simulink model "mcb_pmsm_foc_sensorless_f28379d1"  (R2026a)
settings: Solver=FixedStepDiscrete  StopTime=8  EnableMultiTasking=on
InitFcn:
  | mcb_pmsm_foc_sensorless_f28379d_datascript;
  | mcb_pmsm_foc_sensorless_f28379d_pi_recovery;
  | mcb_pmsm_foc_sensorless_f28379d_fado_init;
  | mcb_pmsm_foc_sensorless_f28379d_fado_tuning;
  | mcb_pmsm_foc_sensorless_f28379d_fado_testprofile_init;
model workspace (MAT data in the model file):
  encoderResolution = 2000
  hallOffset = '0.5'
  indexOffset = 850
  polePairs = '4'
values from neighbouring files (symbols this model uses):
  acceleration = 10000/PU_System.N_base    [mcb_pmsm_foc_sensorless_f28379d_datascript.m]
  dataType = 'single'    [mcb_pmsm_foc_sensorless_f28379d_datascript.m]
  fado_EnableIdAssist = double(fado.EnableIdAssist)    [mcb_pmsm_foc_sensorless_f28379d_fado_init.m]
  fado_EnableVoltagePreprocess = double(fado.EnableVoltagePreprocess)    [mcb_pmsm_foc_sensorless_f28379d_fado_init.m]
  fado_FluxLimit = fado.FluxLimit    [mcb_pmsm_foc_sensorless_f28379d_fado_init.m]
  fado_IBase = fado.IBase    [mcb_pmsm_foc_sensorless_f28379d_fado_init.m]
  fado_IminPU = fado.IminPU    [mcb_pmsm_foc_sensorless_f28379d_fado_init.m]
  fado_Kaf = fado.Kaf    [mcb_pmsm_foc_sensorless_f28379d_fado_init.m]
  fado_Kdf = fado.Kdf    [mcb_pmsm_foc_sensorless_f28379d_fado_init.m]
  fado_LowSpeedHz = fado.LowSpeedHz    [mcb_pmsm_foc_sensorless_f28379d_fado_init.m]
  fado_Lq = fado.Lq    [mcb_pmsm_foc_sensorless_f28379d_fado_init.m]
  fado_LqEstScale = fado.LqEstScale    [mcb_pmsm_foc_sensorless_f28379d_fado_init.m]
  fado_NBase = fado.NBase    [mcb_pmsm_foc_sensorless_f28379d_fado_init.m]
  fado_PolePairs = fado.PolePairs    [mcb_pmsm_foc_sensorless_f28379d_fado_init.m]
  fado_Rs = fado.Rs    [mcb_pmsm_foc_sensorless_f28379d_fado_init.m]
  fado_RsEstScale = fado.RsEstScale    [mcb_pmsm_foc_sensorless_f28379d_fado_init.m]
  fado_T2SFastBandwidthHz = fado.T2SFastBandwidthHz    [mcb_pmsm_foc_sensorless_f28379d_fado_init.m]
  fado_T2SSlowBandwidthHz = fado.T2SSlowBandwidthHz    [mcb_pmsm_foc_sensorless_f28379d_fado_init.m]
  fado_Ts = fado.Ts    [mcb_pmsm_foc_sensorless_f28379d_fado_init.m]
  fado_VAlphaPreprocess = fado.VAlphaPreprocess    [mcb_pmsm_foc_sensorless_f28379d_fado_init.m]
  fado_VBase = fado.VBase    [mcb_pmsm_foc_sensorless_f28379d_fado_init.m]
  fado_VBetaPreprocess = fado.VBetaPreprocess    [mcb_pmsm_foc_sensorless_f28379d_fado_init.m]
  fado_Zeta = fado.Zeta    [mcb_pmsm_foc_sensorless_f28379d_fado_init.m]
  inverter = mcb.updateInverterParameters(pmsm,inverter,target)    [mcb_pmsm_foc_sensorless_f28379d_datascript.m]
  MAX_OL_NEG_SPD = -0.2    [mcb_pmsm_foc_sensorless_f28379d_datascript.m]
  MAX_OL_POS_SPD = 0.2    [mcb_pmsm_foc_sensorless_f28379d_datascript.m]
  MAX_OL_VD_LIMIT = 0.6    [mcb_pmsm_foc_sensorless_f28379d_datascript.m]
  MIN_CL_NEG_SPD = -0.15    [mcb_pmsm_foc_sensorless_f28379d_datascript.m]
  MIN_CL_POS_SPD = 0.15    [mcb_pmsm_foc_sensorless_f28379d_datascript.m]
  MIN_OL_VD_LIMIT = 0.15    [mcb_pmsm_foc_sensorless_f28379d_datascript.m]
  one_sec_tick = uint16(1/Ts_speed)    [mcb_pmsm_foc_sensorless_f28379d_datascript.m]
  PI_params = mcb.calcFOCGains(motor,Ts,Ts_speed,Base=PU_System,PositionObserver=EEMF,SLFeedbackPathDelay=EEMFSLDelay)    [mcb_pmsm_foc_sensorless_f28379d_datascript.m]
  pmsm = mcb.getPMSMParameters('Teknic2310P')    [mcb_pmsm_foc_sensorless_f28379d_datascript.m]
  PU_System = mcb.getPUSystemParameters(pmsm,inverter)    [mcb_pmsm_foc_sensorless_f28379d_datascript.m]
  RAMP_STEP_SIZE = 0.001    [mcb_pmsm_foc_sensorless_f28379d_datascript.m]
  Speed_openLoop_PU = 0.1    [mcb_pmsm_foc_sensorless_f28379d_datascript.m]
  target = mcb.getProcessorParameters('F28379D',PWM_frequency)    [mcb_pmsm_foc_sensorless_f28379d_datascript.m]
  Ts = T_pwm    (= 5e-05)    [mcb_pmsm_foc_sensorless_f28379d_datascript.m]
  Ts_motor = T_pwm/2    (= 2.5e-05)    [mcb_pmsm_foc_sensorless_f28379d_datascript.m]
  Ts_simulink = T_pwm/2    (= 2.5e-05)    [mcb_pmsm_foc_sensorless_f28379d_datascript.m]
  Ts_speed = 10*Ts    (= 0.0005)    [mcb_pmsm_foc_sensorless_f28379d_datascript.m]
  two_sec_tick = uint16(2/Ts_speed)    [mcb_pmsm_foc_sensorless_f28379d_datascript.m]
undefined symbols (not defined in the file or in its folder): bit, DiscIntNeverNeededParam, Down, FADO_TestProfileEnable, GPTRIP1SEL, GPTRIP2SEL, TZ1, TZ2, Up
libraries: mcbcontrolslib x9, c2802xlib x7, mcbeeMathTransformLib x6, simulink x6, c280xlib x5, c2837xDlib x4, slpidlib x3, mcbpositiondecoderlib x3, mcbsensorlessestimatorlib x2, svdschedulerlib x2, svdutilitieslib x1, mcbplantlib x1
(part 3 of 3)

== system mcb_pmsm_foc_sensorless_f28379d1/Current Control/Input Scaling/Calculate position and speed/Flux Observer ==
  InputSignals : Inport
  Action Port : ActionPort  ActionPortLabel=case [ 1 ]:
  Data Store Read1 : DataStoreRead  DataStoreName=Enable  IndexOptions=Index vector (dialog)  Indices=1  OutputSizes=1
  Demux1 : Demux
  Flux Observer : mcbpositiondecoderlib/Flux Observer  DataTypeSelect=off  ParameterBusInput=off  MotorSelection=PMSM  BlockInputUnit=Per-unit  PerUnitVoltage=PU_System.V_base  PerUnitCurrent=PU_System.I_base  PositionSelect=on  FluxSelect=on  TorqueSelect=off  PolePairs=pmsm.p  StatorResistance=pmsm.Rs  StatorDAxisInductance=pmsm.Ld  StatorLeakageInductance=0.0068  RotorLeakageInductance=0.0068  MagnetizingInductance=0.0300  CutoffFreq=FOCutOffFrq  BlockSampleTime=Ts  PositionUnit=Per-unit  PositionDatatype=dataType  FluxUnit=Weber  PerUnitFlux=0.1  FluxDatatype=single  TorqueUnit=Nm  PerUnitTorque=100  TorqueDatatype=single  DataType=0
  IIR Filter4 : mcbcontrolslib/IIR Filter  VariantControl=Low Pass Filter  VariantSelect=Low-pass  FilterConstantInputType=Specify via dialog  Filter_constant=FOSpdFltCoeff  InitialOutput=Specify via dialog  InitialOutputValue=0  ExternalReset=none  advancedSettings=off  Ts=50e-6  cutOff_freq=6.845
  Logical Operator : Logic  Operator=NOT  IconShape=distinctive  AllPortsSameDT=off  OutDataTypeStr=boolean
  Mux2 : Mux  Inputs=2
  Speed Measurement : mcbpositiondecoderlib/Speed Measurement  DiscreteStepInput=off  LastDiscreteStepInput=off  PositionUnit=Per unit  PositionScalingDatatype=uint32  SpeedCalculationMode=Time interval for speed calculation  TempSpeedCalculationMode=Time interval for speed calculation  SampleTimeAsync=Ts  MaximumApplicationSpeed=60000  SpeedResolution=5e-6  DelayLength=10  MaximumMeasurableSpeed=54545.4545  MeasurableSpeedResolution=2.794e-05  SpeedUnit=Per unit based on dialog  TempSpeedUnit=RPM  PerUnitSpeed=PU_System.N_base  SpeedDataType=dataType
  elect2mech : Gain  Gain=1/pmsm.p  RndMeth=Simplest  OutDataTypeStr=Inherit: Same as input
  Position/Speed : Outport
  wires:
  Mux2/1 -> Position/Speed/1
  Speed Measurement/1 -> IIR Filter4/1
  elect2mech/1 -> Mux2/2
  Demux1/3 -> Flux Observer/3  "Ialpha"
  Demux1/4 -> Flux Observer/4  "Ibeta"
  IIR Filter4/1 -> elect2mech/1
  Logical Operator/1 -> Flux Observer/5
  Data Store Read1/1 -> Logical Operator/1
  Flux Observer/1 -> Speed Measurement/1, Mux2/1
  Demux1/1 -> Flux Observer/1
  Demux1/2 -> Flux Observer/2
  InputSignals/1 -> Demux1/1
  Flux Observer/2 -> ?

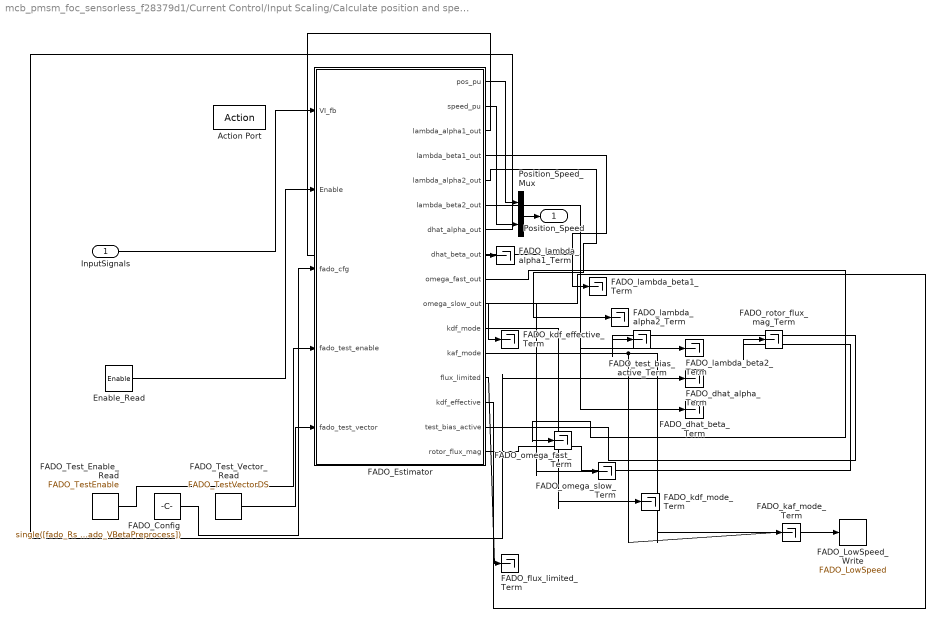
== system mcb_pmsm_foc_sensorless_f28379d1/Current Control/Input Scaling/Calculate position and speed/Frequency_Adaptive_Disturbance_Observer ==
  InputSignals : Inport
  Action Port : ActionPort  ActionPortLabel=case [ 3 ]:
  Enable_Read : DataStoreRead  DataStoreName=Enable  IndexOptions=Index vector (dialog)  Indices=1  OutputSizes=1
  FADO_Config : Constant  Value=single([fado_Rs fado_RsEstScale fado_Lq fado_LqEstScale fado_PolePairs fado_Ts fado_VBase fado_IBase fado_NBase fado_FluxLimit fado_Kdf fado_LowSpeedHz fado_Kaf fado_T2SFastBandwidthHz fado_T2SSlowBandwidthHz fado_Zeta fado_EnableVoltagePreprocess fado_VAlphaPreprocess fado_VBetaPreprocess])
  FADO_Estimator : MATLAB Function  TreatAsAtomicUnit=on
  FADO_LowSpeed_Write : DataStoreWrite  DataStoreName=FADO_LowSpeed  IndexOptions=Index vector (dialog)  Indices=1  OutputSizes=1
  FADO_Test_Enable_Read : DataStoreRead  DataStoreName=FADO_TestEnable  IndexOptions=Index vector (dialog)  Indices=1  OutputSizes=1
  FADO_Test_Vector_Read : DataStoreRead  DataStoreName=FADO_TestVectorDS  IndexOptions=Index vector (dialog)  Indices=1  OutputSizes=1
  FADO_dhat_alpha_Term : Terminator
  FADO_dhat_beta_Term : Terminator
  FADO_flux_limited_Term : Terminator
  FADO_kaf_mode_Term : Terminator
  FADO_kdf_effective_Term : Terminator
  FADO_kdf_mode_Term : Terminator
  FADO_lambda_alpha1_Term : Terminator
  FADO_lambda_alpha2_Term : Terminator
  FADO_lambda_beta1_Term : Terminator
  FADO_lambda_beta2_Term : Terminator
  FADO_omega_fast_Term : Terminator
  FADO_omega_slow_Term : Terminator
  FADO_rotor_flux_mag_Term : Terminator
  FADO_test_bias_active_Term : Terminator
  Position_Speed_Mux : Mux  Inputs=2
  Position_Speed : Outport
  wires:
  FADO_Estimator/16(rotor_flux_mag) -> FADO_rotor_flux_mag_Term/1
  FADO_Estimator/15(test_bias_active) -> FADO_test_bias_active_Term/1
  FADO_Estimator/14(kdf_effective) -> FADO_kdf_effective_Term/1
  FADO_Test_Vector_Read/1 -> FADO_Estimator/5(fado_test_vector)
  FADO_Test_Enable_Read/1 -> FADO_Estimator/4(fado_test_enable)
  FADO_Config/1 -> FADO_Estimator/3(fado_cfg)
  Position_Speed_Mux/1 -> Position_Speed/1
  FADO_Estimator/13(flux_limited) -> FADO_flux_limited_Term/1
  FADO_Estimator/12(kaf_mode) -> FADO_kaf_mode_Term/1, FADO_LowSpeed_Write/1
  FADO_Estimator/11(kdf_mode) -> FADO_kdf_mode_Term/1
  FADO_Estimator/10(omega_slow_out) -> FADO_omega_slow_Term/1
  FADO_Estimator/9(omega_fast_out) -> FADO_omega_fast_Term/1
  FADO_Estimator/8(dhat_beta_out) -> FADO_dhat_beta_Term/1
  FADO_Estimator/7(dhat_alpha_out) -> FADO_dhat_alpha_Term/1
  FADO_Estimator/6(lambda_beta2_out) -> FADO_lambda_beta2_Term/1
  FADO_Estimator/5(lambda_alpha2_out) -> FADO_lambda_alpha2_Term/1
  FADO_Estimator/4(lambda_beta1_out) -> FADO_lambda_beta1_Term/1
  FADO_Estimator/3(lambda_alpha1_out) -> FADO_lambda_alpha1_Term/1
  FADO_Estimator/2(speed_pu) -> Position_Speed_Mux/2
  FADO_Estimator/1(pos_pu) -> Position_Speed_Mux/1
  InputSignals/1 -> FADO_Estimator/1(VI_fb)
  Enable_Read/1 -> FADO_Estimator/2(Enable)

== system mcb_pmsm_foc_sensorless_f28379d1/Current Control/Input Scaling/Calculate position and speed/Sliding Mode Observer ==
  InputSignals : Inport
  Action Port : ActionPort  ActionPortLabel=case [ 0 ]:
  Data Store Read1 : DataStoreRead  DataStoreName=Enable  IndexOptions=Index vector (dialog)  Indices=1  OutputSizes=1
  Demux1 : Demux
  Logical Operator : Logic  Operator=NOT  IconShape=distinctive  AllPortsSameDT=off  OutDataTypeStr=boolean
  Mux : Mux  Inputs=2
  Sliding Mode Observer : mcbsensorlessestimatorlib/Sliding Mode Observer  InputUnit=Per-unit  BlkSampleTime=Ts  StatorResistance=pmsm.Rs  StatorInductance=pmsm.Ld  MaxApplicationSpeed=pmsm.N_base  PolePairs=pmsm.p  MaxStatorVoltage=PU_System.V_base  MaxStatorCurrent=PU_System.I_base  DisturbanceObserverGain=smo.BackEmfObsGain  CurrentObserverGain=smo.CurrentObsGain  CutoffFreq=smo.CutoffFreq  PositionUnit=Per unit  PositionDataType=dataType  SpeedUnit=Per unit  PerUnitSpeed=PU_System.N_base  SpeedDataType=dataType
  Position/Speed : Outport
  wires:
  Mux/1 -> Position/Speed/1
  Demux1/4 -> Sliding Mode Observer/4  "Ibeta"
  Demux1/3 -> Sliding Mode Observer/3  "Ialpha"
  Sliding Mode Observer/1 -> Mux/1
  InputSignals/1 -> Demux1/1
  Data Store Read1/1 -> Logical Operator/1
  Logical Operator/1 -> Sliding Mode Observer/5
  Sliding Mode Observer/2 -> Mux/2
  Demux1/1 -> Sliding Mode Observer/1
  Demux1/2 -> Sliding Mode Observer/2

== system mcb_pmsm_foc_sensorless_f28379d1/Current Control/SCI_Tx/Code Generation/Data_Conditioning_Tx ==
  In1 : Inport
  Data_Type_Fixed_Point : Subsystem  VariantControl=~isequal(dataType,'single')
  Data_Type_Float : Subsystem  VariantControl=isequal(dataType, 'single')
  Data_Log : Outport

== system mcb_pmsm_foc_sensorless_f28379d1/Current Control/SCI_Tx/Code Generation/Data_Logging ==
  note: Fast Serial Data Monitoring (32-bit)
  Data_Log : Inport
  Counter Limited : simulink/Sources/Counter Limited  uplimit=600-1  tsamp=-1
  Data : Subsystem  TreatAsAtomicUnit=on
  End : Subsystem  TreatAsAtomicUnit=on
  If : If  IfExpression=u1 == 0  ElseIfExpressions=u1 == 599
  Merge : Merge  Inputs=3
  Merge1 : Merge  Inputs=3
  Mux : Mux  Inputs=2
  Start : Subsystem  TreatAsAtomicUnit=on
  Width : Width  OutDataTypeMode=All ports same datatype  DataType=uint16
  SCI_Tx : Outport
  wires:
  If/3 -> Data/Action
  Data/1(Data_out) -> Merge/3
  Width/1 -> Data/2(Data_width), Start/2(Data_width), End/2(Data_width)
  Merge/1 -> Mux/1  "SCI_Tx_Data"
  Counter Limited/1 -> If/1
  Start/2(Iteration) -> Merge1/1
  Start/1(Data_out) -> Merge/1
  If/2 -> End/Action
  Merge1/1 -> Mux/2  "SCI_Tx_Iteration"
  If/1 -> Start/Action
  End/1(Data_out) -> Merge/2
  End/2(Iteration) -> Merge1/2
  Data/2(Iteration) -> Merge1/3
  Mux/1 -> SCI_Tx/1
  Data_Log/1 -> Width/1, Start/1(Data), End/1(Data), Data/1(Data)

== system mcb_pmsm_foc_sensorless_f28379d1/Current Control/SCI_Tx/Code Generation/While Iterator Subsystem ==
  Data : Inport
  Iteration : Inport  Port=2
  Add : Sum  Inputs=+-  OutDataTypeStr=Inherit: Same as first input
  Index Vector : MultiPortSwitch  Inputs=1  SaturateOnIntegerOverflow=off  InputSameDT=off
  SCI Transmit : c280xlib/SCI Transmit  sciModule=A  dataHead=''  dataTail=''  frameSize=1  blockingMode=on  outputStatus=off
  While Iterator : WhileIterator  MaxIters=-1  WhileBlockType=do-while  ShowIterationPort=on  OutputDataType=int16
  wires:
  While Iterator/1 -> Add/2, Index Vector/1
  Data/1 -> Index Vector/2
  Index Vector/1 -> SCI Transmit/1
  Add/1 -> While Iterator/1
  Iteration/1 -> Add/1

== system mcb_pmsm_foc_sensorless_f28379d1/Hardware Init/Variant Subsystem/Code Generation/Calculate ADC Offset  ==
  Enable : EnablePort
  Constant : Constant  Value=8
  Constant1 : Constant  Value=inverter.CtSensOffsetMax  OutDataTypeStr=Inherit: Inherit via back propagation
  Constant2 : Constant  Value=inverter.CtSensOffsetMin  OutDataTypeStr=Inherit: Inherit via back propagation
  Divide : Product  Inputs=*/  OutDataTypeStr=uint16
  Divide1 : Product  Inputs=*/  OutDataTypeStr=uint16
  For Iterator Subsystem : Subsystem  TreatAsAtomicUnit=on
  If : If  NumInputs=3  IfExpression=u1 > u3 & u1 < u2
  If Action Subsystem : Subsystem  TreatAsAtomicUnit=on
  If Action Subsystem1 : Subsystem  TreatAsAtomicUnit=on
  If Action Subsystem2 : Subsystem  TreatAsAtomicUnit=on
  If Action Subsystem3 : Subsystem  TreatAsAtomicUnit=on
  If1 : If  NumInputs=3  IfExpression=u1 > u3 & u1 < u2
  wires:
  For Iterator Subsystem/2(Out2) -> Divide1/1
  Divide/1 -> If Action Subsystem/1(In1), If/1
  For Iterator Subsystem/1(Out1) -> Divide/1
  Constant/1 -> Divide1/2, Divide/2
  Divide1/1 -> If Action Subsystem2/1(In1), If1/1
  If/1 -> If Action Subsystem/Action
  If/2 -> If Action Subsystem1/Action
  If1/1 -> If Action Subsystem2/Action
  If1/2 -> If Action Subsystem3/Action
  Constant1/1 -> If1/2, If/2
  Constant2/1 -> If/3, If1/3

== system mcb_pmsm_foc_sensorless_f28379d1/Hardware Init/Variant Subsystem/Code Generation/DRV Enable ==
  note: Enable inverter in CPU1
  In : Inport
  ADC Gain Setting : Subsystem
  Constant : Constant  Value=inverter.EnableLogic
  Digital Output : c2837xDlib/Digital Output  Priority=10  GPIO_Number=GPIO120~GPIO127  GPIO_Bit0=off  GPIO_BIT0_Toggle=off  GPIO_Bit1=off  GPIO_BIT1_Toggle=off  GPIO_Bit2=off  GPIO_BIT2_Toggle=off  GPIO_Bit3=off  GPIO_BIT3_Toggle=off  GPIO_Bit4=on  GPIO_BIT4_Toggle=off  GPIO_Bit5=off  GPIO_BIT5_Toggle=off  GPIO_Bit6=off  GPIO_BIT6_Toggle=off  GPIO_Bit7=off  GPIO_BIT7_Toggle=off
  Digital Output1 : c2837xDlib/Digital Output  Priority=10  GPIO_Number=GPIO16~GPIO23  GPIO_Bit0=off  GPIO_BIT0_Toggle=off  GPIO_Bit1=off  GPIO_BIT1_Toggle=off  GPIO_Bit2=off  GPIO_BIT2_Toggle=off  GPIO_Bit3=off  GPIO_BIT3_Toggle=off  GPIO_Bit4=off  GPIO_BIT4_Toggle=off  GPIO_Bit5=off  GPIO_BIT5_Toggle=off  GPIO_Bit6=on  GPIO_BIT6_Toggle=off  GPIO_Bit7=off  GPIO_BIT7_Toggle=off
  Inverter Enable : Constant  OutDataTypeStr=uint16  SampleTime=-1
  NOT : Logic  Operator=NOT  IconShape=distinctive  AllPortsSameDT=off  OutDataTypeStr=boolean
  RunTimeMeasurement : Constant  OutDataTypeStr=uint16  SampleTime=-1
  Switch : Switch  Criteria=u2 > Threshold  SaturateOnIntegerOverflow=off  InputSameDT=off
  wires:
  RunTimeMeasurement/1 -> Digital Output1/1
  NOT/1 -> Switch/3  "Active low logic for inverter enable"
  Inverter Enable/1 -> Switch/1, NOT/1  "Active high logic for inverter enable"
  Constant/1 -> ADC Gain Setting/Enable, Switch/2
  Switch/1 -> Digital Output/1
  In/1 -> ADC Gain Setting/1(In1)

== system mcb_pmsm_foc_sensorless_f28379d1/Hardware Init/Variant Subsystem/Code Generation/Default ADC Offset ==
  Enable : EnablePort
  Constant : Constant  Value=inverter.CtSensAOffset  OutDataTypeStr=Inherit: Inherit via back propagation
  Constant1 : Constant  Value=inverter.CtSensBOffset  OutDataTypeStr=Inherit: Inherit via back propagation
  Data Store Write1 : DataStoreWrite  DataStoreName=IaOffset  IndexOptions=Index vector (dialog)  Indices=1  OutputSizes=1
  Data Store Write2 : DataStoreWrite  DataStoreName=IbOffset  IndexOptions=Index vector (dialog)  Indices=1  OutputSizes=1
  wires:
  Constant/1 -> Data Store Write1/1
  Constant1/1 -> Data Store Write2/1

== system mcb_pmsm_foc_sensorless_f28379d1/Serial Receive/SCI_Rx/Code Generation/Data_Type_Fixed_Point ==
  SCI Receive : c280xlib/SCI Receive  sciModule=A  dataHead=''  headerCheckMaxCount=16  dataTail=''  dataType=uint32  dataLenOptions=Length via dialog  dataDim=2  maxDataLength=1  initValue=0  errOption=Output the last received value  errValue=0  sampleTime=-1  blockingMode=on  timeOut=0.00875  outputStatus=off
  Data : Outport
  wires:
  SCI Receive/1 -> Data/1

== system mcb_pmsm_foc_sensorless_f28379d1/Serial Receive/SCI_Rx/Code Generation/Data_Type_Float ==
  SCI Receive : c280xlib/SCI Receive  sciModule=A  dataHead=''  headerCheckMaxCount=16  dataTail=''  dataType=single  dataLenOptions=Length via dialog  dataDim=2  maxDataLength=1  initValue=0  errOption=Output the last received value  errValue=0  sampleTime=-1  blockingMode=on  timeOut=0.00875  outputStatus=off
  Data : Outport
  wires:
  SCI Receive/1 -> Data/1

== system mcb_pmsm_foc_sensorless_f28379d1/Serial Receive/SCI_Rx/Simulation/Data_Conditioning_Tx ==
  In1 : Inport
  In2 : Inport  Port=2
  Data_Type_Fixed_Point : Subsystem  VariantControl=~isequal(dataType, 'single')
  Data_Type_Float : Subsystem  VariantControl=isequal(dataType, 'single')
  Data : Outport

== system mcb_pmsm_foc_sensorless_f28379d1/Serial Receive/SCI_Rx/Simulation/Parse ==
  Enable_PWM : Inport
  Debug_signals : Inport  Port=2
  Bitwise Operator : simulink/Logic and Bit Operations/Bitwise Operator  logicop=AND  UseBitMask=on  BitMask=hex2dec('0001')  BitMaskRealWorld=Stored Integer
  Bitwise Operator1 : simulink/Logic and Bit Operations/Bitwise Operator  logicop=AND  UseBitMask=on  BitMask=hex2dec('00F0')  BitMaskRealWorld=Stored Integer
  Shift Arithmetic1 : ArithShift  BitShiftNumber=-4
  Sum : Sum
  Data : Outport
  wires:
  Bitwise Operator/1 -> Sum/1
  Debug_signals/1 -> Shift Arithmetic1/1
  Sum/1 -> Data/1
  Shift Arithmetic1/1 -> Bitwise Operator1/1
  Enable_PWM/1 -> Bitwise Operator/1
  Bitwise Operator1/1 -> Sum/2

== system mcb_pmsm_foc_sensorless_f28379d1/Current Control/Closed Loop/Open_Loop_Control/Accumulate1/Subsystem ==
  Input : Inport
  Enable : EnablePort
  Out1 : Outport  InitialOutput=0
  wires:
  Input/1 -> Out1/1

== system mcb_pmsm_foc_sensorless_f28379d1/Current Control/Input Scaling/Calculate Phase Currents/Data_Type/Data_Type_Fixed_Point ==
  In1 : Inport
  Data Type Conversion : DataTypeConversion  OutDataTypeStr=fixdt(1,32,17)  ConvertRealWorld=Stored Integer (SI)  RndMeth=Simplest  SaturateOnIntegerOverflow=off
  Data Type Conversion1 : DataTypeConversion  OutDataTypeStr=dataType  RndMeth=Simplest  SaturateOnIntegerOverflow=off
  Q17 per unit conversion : ArithShift  BitShiftNumber=-6
  Iab_meas_PU : Outport
  wires:
  In1/1 -> Q17 per unit conversion/1
  Data Type Conversion1/1 -> Iab_meas_PU/1
  Data Type Conversion/1 -> Data Type Conversion1/1
  Q17 per unit conversion/1 -> Data Type Conversion/1

== system mcb_pmsm_foc_sensorless_f28379d1/Current Control/Input Scaling/Calculate Phase Currents/Data_Type/Data_Type_Float ==
  In1 : Inport
  Get ADC Voltage : Gain  Gain=target.ADC_Vref /target.ADC_MaxCount  OutDataTypeStr=dataType  RndMeth=Simplest
  Get Currents : Gain  Gain=1/inverter.ISenseVoltPerAmp  RndMeth=Simplest  OutDataTypeStr=Inherit: Same as input
  PU_Conversion : Gain  Gain=1/PU_System.I_base  RndMeth=Simplest  OutDataTypeStr=Inherit: Same as input
  Iab_meas_PU : Outport
  wires:
  Get ADC Voltage/1 -> Get Currents/1
  Get Currents/1 -> PU_Conversion/1
  PU_Conversion/1 -> Iab_meas_PU/1
  In1/1 -> Get ADC Voltage/1

== system mcb_pmsm_foc_sensorless_f28379d1/Current Control/SCI_Tx/Code Generation/Data_Conditioning_Tx/Data_Type_Fixed_Point ==
  In1 : Inport
  Data Type Conversion : DataTypeConversion  OutDataTypeStr=fixdt(1,32,28)  RndMeth=Simplest  SaturateOnIntegerOverflow=off
  Data Type Conversion3 : DataTypeConversion  OutDataTypeStr=uint32  ConvertRealWorld=Stored Integer (SI)  RndMeth=Simplest  SaturateOnIntegerOverflow=off
  Data_Log : Outport
  wires:
  In1/1 -> Data Type Conversion/1
  Data Type Conversion3/1 -> Data_Log/1
  Data Type Conversion/1 -> Data Type Conversion3/1

== system mcb_pmsm_foc_sensorless_f28379d1/Current Control/SCI_Tx/Code Generation/Data_Conditioning_Tx/Data_Type_Float ==
  In1 : Inport
  Byte Pack : svdutilitieslib/Byte Pack  maskPackedDataType=uint32  datatypes={'single'}  byteAlign=4  blockPlatform=tic2000
  Data_Log : Outport
  wires:
  Byte Pack/1 -> Data_Log/1
  In1/1 -> Byte Pack/1

== system mcb_pmsm_foc_sensorless_f28379d1/Current Control/SCI_Tx/Code Generation/Data_Logging/Data ==
  Data : Inport
  Data_width : Inport  Port=2
  Action Port : ActionPort  ActionPortLabel=else
  Dummy : Constant  Value=hex2dec('0000')  OutDataTypeStr=uint32
  Mux : Mux  Inputs=2
  Data_out : Outport  VectorParamsAs1DForOutWhenUnconnected=off
  Iteration : Outport  Port=2  VectorParamsAs1DForOutWhenUnconnected=off
  wires:
  Data_width/1 -> Iteration/1
  Data/1 -> Mux/1
  Dummy/1 -> Mux/2
  Mux/1 -> Data_out/1

== system mcb_pmsm_foc_sensorless_f28379d1/Current Control/SCI_Tx/Code Generation/Data_Logging/End ==
  Data : Inport
  Data_width : Inport  Port=2
  Action Port : ActionPort  ActionPortLabel=elseif(u1 == 599)
  Bias : Bias  Bias=1  SaturateOnIntegerOverflow=off
  End : Constant  Value=hex2dec('45454545')  OutDataTypeStr=uint32
  Mux : Mux  Inputs=2
  Data_out : Outport  VectorParamsAs1DForOutWhenUnconnected=off
  Iteration : Outport  Port=2  VectorParamsAs1DForOutWhenUnconnected=off
  wires:
  Data/1 -> Mux/1
  Data_width/1 -> Bias/1
  Bias/1 -> Iteration/1
  End/1 -> Mux/2
  Mux/1 -> Data_out/1

== system mcb_pmsm_foc_sensorless_f28379d1/Current Control/SCI_Tx/Code Generation/Data_Logging/Start ==
  Data : Inport
  Data_width : Inport  Port=2
  Action Port : ActionPort  ActionPortLabel=if(u1 == 0)
  Bias : Bias  Bias=1  SaturateOnIntegerOverflow=off
  Mux : Mux  Inputs=2
  Start : Constant  Value=hex2dec('53535353')  OutDataTypeStr=uint32
  Data_out : Outport  VectorParamsAs1DForOutWhenUnconnected=off
  Iteration : Outport  Port=2  VectorParamsAs1DForOutWhenUnconnected=off
  wires:
  Data/1 -> Mux/2
  Data_width/1 -> Bias/1
  Bias/1 -> Iteration/1
  Start/1 -> Mux/1
  Mux/1 -> Data_out/1

== system mcb_pmsm_foc_sensorless_f28379d1/Hardware Init/Variant Subsystem/Code Generation/Calculate ADC Offset /For Iterator Subsystem ==
  ADC_B2 : c2802xlib/ADC  Priority=20  blkParamProc=C2000_Type4  ADCModule=B  samplingMode=Single sample mode  ADCResolution=12-bit (Single-ended input)  ADC29xResolution=12-bit  ADCMode=Single-ended input  useSOC1=SOC2  useSOC2=SOC0_SOC1  SOCAcquisitionWindow=15  SOCTriggerSource=Software  SOCInterruptTrigger=No ADCINT  Ts=-1  dType=uint16  postInterrupt=off  interruptSel=ADCINT1  ADCINTContinuous=on  endma=off  chdma=1  conv1=ADCINA0  conv2=ADCINA0 and ADCINB0  conv1_Type4=ADCIN2  conv2_Type4=ADCIN0 and ADCIN1
  ADC_C2 : c2802xlib/ADC  Priority=20  blkParamProc=C2000_Type4  ADCModule=C  samplingMode=Single sample mode  ADCResolution=12-bit (Single-ended input)  ADC29xResolution=12-bit  ADCMode=Single-ended input  useSOC1=SOC2  useSOC2=SOC0_SOC1  SOCAcquisitionWindow=15  SOCTriggerSource=Software  SOCInterruptTrigger=No ADCINT  Ts=-1  dType=uint16  postInterrupt=off  interruptSel=ADCINT1  ADCINTContinuous=on  endma=off  chdma=1  conv1=ADCINA0  conv2=ADCINA0 and ADCINB0  conv1_Type4=ADCIN2  conv2_Type4=ADCIN0 and ADCIN1
  For Iterator : ForIterator  IterationLimit=16  IterationVariableDataType=uint16
  If : If  IfExpression=u1 > 8  ShowElse=off
  If Action Subsystem : Subsystem  TreatAsAtomicUnit=on
  Out1 : Outport
  Out2 : Outport  Port=2
  wires:
  For Iterator/1 -> If/1
  ADC_C2/1 -> If Action Subsystem/1(In1)
  ADC_B2/1 -> If Action Subsystem/2(In2)
  If Action Subsystem/1(Out1) -> Out1/1
  If Action Subsystem/2(Out2) -> Out2/1
  If/1 -> If Action Subsystem/Action

== system mcb_pmsm_foc_sensorless_f28379d1/Hardware Init/Variant Subsystem/Code Generation/Calculate ADC Offset /If Action Subsystem ==
  In1 : Inport
  Action Port : ActionPort  ActionPortLabel=if(u1 > u3 & u1 < u2)
  Data Store Write1 : DataStoreWrite  DataStoreName=IaOffset  IndexOptions=Index vector (dialog)  Indices=1  OutputSizes=1
  wires:
  In1/1 -> Data Store Write1/1

== system mcb_pmsm_foc_sensorless_f28379d1/Hardware Init/Variant Subsystem/Code Generation/Calculate ADC Offset /If Action Subsystem1 ==
  Action Port : ActionPort  ActionPortLabel=else
  Constant : Constant  Value=inverter.CtSensAOffset  OutDataTypeStr=Inherit: Inherit via back propagation
  Data Store Write1 : DataStoreWrite  DataStoreName=IaOffset  IndexOptions=Index vector (dialog)  Indices=1  OutputSizes=1
  wires:
  Constant/1 -> Data Store Write1/1

== system mcb_pmsm_foc_sensorless_f28379d1/Hardware Init/Variant Subsystem/Code Generation/Calculate ADC Offset /If Action Subsystem2 ==
  In1 : Inport
  Action Port : ActionPort  ActionPortLabel=if(u1 > u3 & u1 < u2)
  Data Store Write2 : DataStoreWrite  DataStoreName=IbOffset  IndexOptions=Index vector (dialog)  Indices=1  OutputSizes=1
  wires:
  In1/1 -> Data Store Write2/1

== system mcb_pmsm_foc_sensorless_f28379d1/Hardware Init/Variant Subsystem/Code Generation/Calculate ADC Offset /If Action Subsystem3 ==
  Action Port : ActionPort  ActionPortLabel=else
  Constant1 : Constant  Value=inverter.CtSensBOffset  OutDataTypeStr=Inherit: Inherit via back propagation
  Data Store Write2 : DataStoreWrite  DataStoreName=IbOffset  IndexOptions=Index vector (dialog)  Indices=1  OutputSizes=1
  wires:
  Constant1/1 -> Data Store Write2/1

== system mcb_pmsm_foc_sensorless_f28379d1/Hardware Init/Variant Subsystem/Code Generation/DRV Enable/ADC Gain Setting ==
  In1 : Inport
  Enable : EnablePort
  Demux : Demux  Outputs=2
  Display : Display
      settings: Format=hex (Stored Integer)
  Display1 : Display
      settings: Format=hex (Stored Integer)
  SPI Master Transfer : c280xlib/SPI Controller Transfer  SPISelect=SPI_A  ClockPolarity=Rising_edge  ClockPhase=No_delay  SPIModule=uint32(0)  Mode=Master  BusSpeed=uint32(1000000)  FirstBitToTransfer=Most significant bit (MSB)  ClockMode=0  BlockFunction=Transfer  EnableRegisterAddress=off  RegisterAddress=0  OutputDataType=int8  OutputDataLength=1  DataBits=16  UseCustomSSPin=Provided by the SPI peripheral  ActiveLowSSPin=Active low  Pin=61
  SPI Master Transfer1 : c280xlib/SPI Controller Transfer  SPISelect=SPI_A  ClockPolarity=Rising_edge  ClockPhase=No_delay  SPIModule=uint32(0)  Mode=Master  BusSpeed=uint32(1000000)  FirstBitToTransfer=Most significant bit (MSB)  ClockMode=0  BlockFunction=Transfer  EnableRegisterAddress=off  RegisterAddress=0  OutputDataType=int8  OutputDataLength=1  DataBits=16  UseCustomSSPin=Provided by the SPI peripheral  ActiveLowSSPin=Active low  Pin=61
  wires:
  Demux/2 -> SPI Master Transfer1/1
  SPI Master Transfer/1 -> Display/1
  SPI Master Transfer1/1 -> Display1/1
  Demux/1 -> SPI Master Transfer/1
  In1/1 -> Demux/1

== system mcb_pmsm_foc_sensorless_f28379d1/Serial Receive/SCI_Rx/Simulation/Data_Conditioning_Tx/Data_Type_Fixed_Point ==
  In1 : Inport
  In2 : Inport  Port=2
  Data Type Conversion : DataTypeConversion  OutDataTypeStr=fixdt(1,32,28)  RndMeth=Simplest  SaturateOnIntegerOverflow=off
  Data Type Conversion1 : DataTypeConversion  OutDataTypeStr=uint32  RndMeth=Simplest  SaturateOnIntegerOverflow=off
  Data Type Conversion3 : DataTypeConversion  OutDataTypeStr=uint32  ConvertRealWorld=Stored Integer (SI)  RndMeth=Simplest  SaturateOnIntegerOverflow=off
  Mux : Mux  Inputs=2
  Data : Outport
  wires:
  In1/1 -> Data Type Conversion/1
  Data Type Conversion3/1 -> Mux/1
  Data Type Conversion/1 -> Data Type Conversion3/1
  In2/1 -> Data Type Conversion1/1
  Data Type Conversion1/1 -> Mux/2
  Mux/1 -> Data/1

== system mcb_pmsm_foc_sensorless_f28379d1/Serial Receive/SCI_Rx/Simulation/Data_Conditioning_Tx/Data_Type_Float ==
  In1 : Inport
  In2 : Inport  Port=2
  Data Type Conversion2 : DataTypeConversion  OutDataTypeStr=single  RndMeth=Simplest  SaturateOnIntegerOverflow=off
  Mux : Mux  Inputs=2
  Data : Outport
  wires:
  In1/1 -> Mux/1
  Mux/1 -> Data/1
  In2/1 -> Data Type Conversion2/1
  Data Type Conversion2/1 -> Mux/2

== system mcb_pmsm_foc_sensorless_f28379d1/Hardware Init/Variant Subsystem/Code Generation/Calculate ADC Offset /For Iterator Subsystem/If Action Subsystem ==
  In1 : Inport
  In2 : Inport  Port=2
  Action Port : ActionPort  ActionPortLabel=if(u1 > 8)
  Memory : Memory  InheritSampleTime=on
  Memory1 : Memory  InheritSampleTime=on
  Sum : Sum
  Sum1 : Sum
  Out1 : Outport
  Out2 : Outport  Port=2
  wires:
  In1/1 -> Sum/1
  Sum/1 -> Out1/1, Memory/1
  In2/1 -> Sum1/1
  Memory/1 -> Sum/2
  Sum1/1 -> Out2/1, Memory1/1
  Memory1/1 -> Sum1/2

== matlab function mcb_pmsm_foc_sensorless_f28379d1/Current Control/Input Scaling/Calculate position and speed/MATLAB Function1 ==
  data: theta_in input; omega_hat output; state input; Ts input; bandwidth input; theta_filtered output; state output
%% ========================================================================
%  T2S (Type 2 System) 函数 - 用于速度和角度估计
%  类似于锁相环 (PLL)
% =========================================================================

function [omega_hat, theta_filtered, state] = T2S(theta_in, state, Ts, bandwidth)
% state: [integrator1, integrator2, prev_theta]

if isempty(state)
    state = [0, 0, 0];
end

int1 = state(1);  % 第一个积分器输出
int2 = state(2);  % 第二个积分器输出 (滤波后的角度)

% T2S增益 (根据带宽设置)
Kp = 2 * bandwidth;
Ki = bandwidth^2;

% 角度误差
theta_error = theta_in - int2;

% 状态更新
d_int1 = Ki * theta_error;
int1 = int1 + d_int1 * Ts;
 
d_int2 = Kp * theta_error + int1;
int2 = int2 + d_int2 * Ts;

% 输出
omega_hat = int1 + Kp * theta_error;
theta_filtered = int2;

% 更新状态
state = [int1, int2, theta_in];
endfunction y = fcn(u)

y = u;

== matlab function mcb_pmsm_foc_sensorless_f28379d1/Current Control/Input Scaling/Calculate position and speed/MATLAB Function ==
  data: lambda_alpha_in input; lambda_alpha_out output; lambda_beta_in input; i_alpha input; i_beta input; omega_f input; Ts input; params input; lambda_beta_out output; D_alpha_out output; D_beta_out output
%% ========================================================================
%  独立的干扰观测器函数 (可直接用于实际控制)
%  Frequency-Adaptive Disturbance Observer (FADO) Function
% =========================================================================

function [lambda_alpha_out, lambda_beta_out, D_alpha_out, D_beta_out] = ...
    FrequencyAdaptiveDOB(lambda_alpha_in, lambda_beta_in, ...
                          i_alpha, i_beta, omega_f, Ts, params)
    
    % 静态变量用于存储状态
    persistent lambda_alpha_prev lambda_beta_prev D_alpha_prev D_beta_prev
    
    % 初始化
    if isempty(lambda_alpha_prev)
        lambda_alpha_prev = 0;
        lambda_lambda_beta_prev = 0;
        D_alpha_prev = 0;
        D_beta_prev = 0;
    end
    
    % 计算观测器增益 (方程16)
    abs_omega = abs(omega_f);
    
    if abs_omega < 0.001
        % 低速时冻结观测器
        D_alpha_out = D_alpha_prev;
        D_beta_out = D_beta_prev;
        lambda_alpha_out = lambda_alpha_in;
        lambda_beta_out = lambda_beta_in;
        return;
    end
    
    % 计算通量变化率
    d_lambda_alpha = (lambda_alpha_in - lambda_alpha_prev) / Ts;
    d_lambda_beta = (lambda_beta_in - lambda_beta_prev) / Ts;
    
    % 更新干扰估计 (方程17的离散实现)
    omega_sq = omega_f^2;
    two_abs_omega = 2 * abs_omega;
    
    D_alpha_new = D_alpha_prev + Ts * (omega_sq * lambda_alpha_in - ...
                        omega_f * d_lambda_beta - two_abs_omega * D_alpha_prev);
                    
    D_beta_new = D_beta_prev + Ts * (omega_f * d_lambda_alpha + ...
                        omega_sq * lambda_beta_in - two_abs_omega * D_beta_prev);
    
    % 更新状态
    lambda_alpha_prev = lambda_alpha_in;
    lambda_beta_prev = lambda_beta_in;
    D_alpha_prev = D_alpha_new;
    D_beta_prev = D_beta_new;
    
    % 输出补偿后的通量 (方程20)
    lambda_alpha_out = lambda_alpha_in - D_alpha_new;
    lambda_beta_out = lambda_beta_in - D_beta_new;
    D_alpha_out = D_alpha_new;
    D_beta_out = D_beta_new;
end

== stateflow chart mcb_pmsm_foc_sensorless_f28379d1/State Machine Handler/State Machine OL - CL ==
  state Halt
    entry:
    Enable=false;
    SpdRef=0;
    EnClosedLoop=false;
  state RunMode
    state PositiveSpeedRun
      state OpenLoopPosRun
        during:
        if(SpdCmd>MAX_OL_POS_SPD)
        SpdRef=MAX_OL_POS_SPD;
        else
        SpdRef=SpdCmd;
        end
      state PreparePosCLSwitch
        entry:
        Id0_out=Id0_in;
        SpdRef=MAX_OL_POS_SPD;
      state TransferToPosClosedLoop
        entry:
        EnClosedLoop=true;
        Id0_out=Id0_in;
        during:
        Id0_out = ComputeId0(Id0_out,RAMP_STEP_SIZE);
      state TransferToOpenLoop
        entry:
        SpdRef=MAX_OL_POS_SPD*1.03;
      state ClosedLoopPosRun
        entry:
        SpdRef=SpdCmd;
        Id0_out=0;
        during:
        if(EstimatorSelector==3)
        Enable=true;
        EnClosedLoop=true;
        SpdRef=SpdCmd;
        Id0_out=0;
        else
        SpdRef=SpdCmd;
        end
      OpenLoopPosRun -> (junction 118)
      (junction 118) -> (junction 94) [order 1] : [SpdCmd>MAX_OL_POS_SPD]
      (junction 94) -> PreparePosCLSwitch [order 2] : [SpdRef<MAX_OL_POS_SPD]
      (junction 94) -> TransferToPosClosedLoop [order 1] : [SpdRef>=MAX_OL_POS_SPD]
      PreparePosCLSwitch -> TransferToPosClosedLoop : after(one_sec_tick,tick)
      TransferToPosClosedLoop -> ClosedLoopPosRun : after(two_sec_tick,tick)[Id0_out<=RAMP_STEP_SIZE]
      ClosedLoopPosRun -> TransferToOpenLoop : [SpdCmd<MIN_CL_POS_SPD && EstimatorSelector~=3]
    state InitOpenLoopRun
      entry:
      Enable=true;
      EnClosedLoop=false;
      during:
      if(SpdCmd>MAX_OL_POS_SPD)
      SpdRef=MAX_OL_POS_SPD;
      elseif (SpdCmd<MAX_OL_NEG_SPD)
      SpdRef=MAX_OL_NEG_SPD;
      else
      SpdRef=SpdCmd;
      end
      Id0_out=Id0_in;
    state Id0_out = ComputeId0(Id0_in,RAMP_STEP_SIZE) [function]
    state NegativeSpeedRun
      state OpenLoopNegRun
        during:
        if(SpdCmd<MAX_OL_NEG_SPD)
        SpdRef=MAX_OL_NEG_SPD;
        else
        SpdRef=SpdCmd;
        end
      state TransferToNegClosedLoop
        entry:
        EnClosedLoop=true;
        Id0_out=Id0_in;
        during:
        Id0_out = ComputeId0(Id0_out,RAMP_STEP_SIZE);
      state PrepareNegCLSwitch
        entry:
        Id0_out=Id0_in;
        SpdRef=MAX_OL_NEG_SPD;
      state TransferToOpenLoop_NEG
        entry:
        SpdRef=MAX_OL_NEG_SPD*1.03;
      state ClosedLoopRun_NEG
        entry:
        SpdRef=SpdCmd;
        Id0_out=0;
        during:
        if(EstimatorSelector==3)
        Enable=true;
        EnClosedLoop=true;
        SpdRef=SpdCmd;
        Id0_out=0;
        else
        SpdRef=SpdCmd;
        end
      OpenLoopNegRun -> (junction 121)
      (junction 121) -> (junction 124) [order 2] : [SpdCmd<MAX_OL_NEG_SPD]
      (junction 124) -> PrepareNegCLSwitch [order 1] : [SpdRef>MAX_OL_NEG_SPD]
      (junction 124) -> TransferToNegClosedLoop [order 2] : [SpdRef<=MAX_OL_NEG_SPD]
      PrepareNegCLSwitch -> TransferToNegClosedLoop : after(one_sec_tick,tick)
      TransferToNegClosedLoop -> ClosedLoopRun_NEG : after(two_sec_tick,tick)[Id0_out<=RAMP_STEP_SIZE]
      ClosedLoopRun_NEG -> TransferToOpenLoop_NEG : [SpdCmd>MIN_CL_NEG_SPD && EstimatorSelector~=3]
    state FADO_ZeroSpeed_Hold_Init
      entry:
      Enable=true;
      EnClosedLoop=true;
      SpdRef=0;
      Id0_out=0;
      during:
      Enable=true;
      EnClosedLoop=true;
      SpdRef=0;
      Id0_out=0;
    (junction 118) -> OpenLoopNegRun [order 2] : [SpdCmd<0]
    InitOpenLoopRun -> OpenLoopPosRun [order 1] : [SpdCmd > 0]
    (junction 121) -> OpenLoopPosRun [order 1] : [SpdCmd>0]
    (default) -> InitOpenLoopRun
    TransferToOpenLoop -> InitOpenLoopRun : after(one_sec_tick,tick)
    InitOpenLoopRun -> FADO_ZeroSpeed_Hold_Init [order 3] : [EstimatorSelector==3 && SpdCmd==0]
    FADO_ZeroSpeed_Hold_Init -> InitOpenLoopRun : [SpdCmd~=0]
    TransferToOpenLoop_NEG -> InitOpenLoopRun : after(one_sec_tick,tick)
    InitOpenLoopRun -> OpenLoopNegRun [order 2] : [SpdCmd<0]
  (default) -> Halt
  RunMode -> Halt : [Start==false || (SpdCmd==0 && EstimatorSelector~=3)]
  Halt -> RunMode : [Start==true && (SpdCmd~=0 || EstimatorSelector==3)]
  data: Id0_in function_input dataType size=1; RAMP_STEP_SIZE function_input dataType size=1; Id0_out function_output; Enable output; EnClosedLoop output; SpdRef output; Start input; SpdCmd input; Id0_out output dataType; Id0_in input; one_sec_tick parameter; two_sec_tick parameter; RAMP_STEP_SIZE parameter dataType; MAX_OL_NEG_SPD parameter dataType; MIN_CL_NEG_SPD parameter dataType; MIN_CL_POS_SPD parameter dataType; MAX_OL_POS_SPD parameter dataType; EstimatorSelector input uint32

== matlab function mcb_pmsm_foc_sensorless_f28379d1/Current Control/Input Scaling/Calculate position and speed/MATLAB Function2 ==
  data: lambda_alpha input; theta_est output; lambda_beta input; i_alpha input; i_beta input; Lq input
%% ========================================================================
%  转子角度估计函数 (方程6)
% =========================================================================

function theta_est = EstimateRotorAngle(lambda_alpha, lambda_beta, i_alpha, i_beta, Lq)
    % 方程6: θr = tan⁻¹((λβ - Lq·iβ)/(λα - Lq·iα))
    
    % 补偿q轴电感压降
    lambda_alpha_comp = lambda_alpha - Lq * i_alpha;
    lambda_beta_comp = lambda_beta - Lq * i_beta;
    
    % 计算角度
    theta_est = atan2(lambda_beta_comp, lambda_alpha_comp);
end

== matlab function mcb_pmsm_foc_sensorless_f28379d1/Current Control/Input Scaling/Calculate position and speed/MATLAB Function3 ==
  data: lambda_alpha input; lambda_alpha_lim output; lambda_beta input; i_alpha input; i_beta input; Lq input; lambda_max input; kaf input; Ts input; lambda_beta_lim output; flux_limited output
%% ========================================================================
%  低速通量限幅器 (图7)
% =========================================================================

function [lambda_alpha_lim, lambda_beta_lim, flux_limited] = ...
    FluxLimiter(lambda_alpha, lambda_beta, i_alpha, i_beta, Lq, ...
                lambda_max, kaf, Ts)
    
    % 计算转子磁通 (方程5)
    lambda_alpha_r = lambda_alpha - Lq * i_alpha;
    lambda_beta_r = lambda_beta - Lq * i_beta;
    
    % 计算磁通幅值
    lambda_mag = sqrt(lambda_alpha_r^2 + lambda_beta_r^2);
    
    % 检查是否需要限幅
    if lambda_mag > lambda_max
        % 应用限幅
        scale = lambda_max / lambda_mag;
        lambda_alpha_r_lim = lambda_alpha_r * scale;
        lambda_beta_r_lim = lambda_beta_r * scale;
        
        % 反积分饱和 (方程25)
        lambda_alpha_lim = lambda_alpha + kaf * (lambda_alpha_r_lim - lambda_alpha_r) * Ts;
        lambda_beta_lim = lambda_beta + kaf * (lambda_beta_r_lim - lambda_beta_r) * Ts;
        flux_limited = true;
    else
        lambda_alpha_lim = lambda_alpha;
        lambda_beta_lim = lambda_beta;
        flux_limited = false;
    end
end

== matlab function mcb_pmsm_foc_sensorless_f28379d1/Current Control/Input Scaling/Calculate position and speed/Frequency_Adaptive_Disturbance_Observer/FADO_Estimator ==
  data: VI_fb input single size=4; pos_pu output single size=1; Enable input boolean size=1; speed_pu output single size=1; lambda_alpha1_out output single size=1; lambda_beta1_out output single size=1; lambda_alpha2_out output single size=1; lambda_beta2_out output single size=1; dhat_alpha_out output single size=1; dhat_beta_out output single size=1; omega_fast_out output single size=1; omega_slow_out output single size=1; kdf_mode output boolean size=1; kaf_mode output boolean size=1; flux_limited output boolean size=1; fado_cfg input single size=19; fado_test_enable input; fado_test_vector input; kdf_effective output; test_bias_active output; rotor_flux_mag output
function [pos_pu, speed_pu, lambda_alpha1_out, lambda_beta1_out, lambda_alpha2_out, lambda_beta2_out, dhat_alpha_out, dhat_beta_out, omega_fast_out, omega_slow_out, kdf_mode, kaf_mode, flux_limited, kdf_effective, test_bias_active, rotor_flux_mag] = FADO_Estimator(VI_fb, Enable, fado_cfg, fado_test_enable, fado_test_vector)
% FADO observer with a simulation-only paper-reproduction input.
persistent lambda_alpha1 lambda_beta1 lambda_alpha_hat lambda_beta_hat
persistent dhat_alpha dhat_beta theta_fast theta_slow omega_fast omega_slow
rs_nom = double(fado_cfg(1));
rs_scale = double(fado_cfg(2));
lq_nom = double(fado_cfg(3));
lq_scale = double(fado_cfg(4));
pole_pairs = double(fado_cfg(5));
Ts_fado = double(fado_cfg(6));
v_base = double(fado_cfg(7));
i_base = double(fado_cfg(8));
n_base = double(fado_cfg(9));
flux_limit = double(fado_cfg(10));
kdf = double(fado_cfg(11));
low_speed_hz = double(fado_cfg(12));
kaf = double(fado_cfg(13));
fast_bandwidth_hz = double(fado_cfg(14));
slow_bandwidth_hz = double(fado_cfg(15));
zeta = double(fado_cfg(16));
enable_voltage_preprocess = fado_cfg(17) ~= 0;
v_alpha_preprocess = double(fado_cfg(18));
v_beta_preprocess = double(fado_cfg(19));
test_profile_enable = fado_test_enable ~= 0;

if isempty(lambda_alpha1)
    lambda_alpha1 = 0.0;
    lambda_beta1 = 0.0;
    lambda_alpha_hat = 0.0;
    lambda_beta_hat = 0.0;
    dhat_alpha = 0.0;
    dhat_beta = 0.0;
    theta_fast = 0.0;
    theta_slow = 0.0;
    omega_fast = 0.0;
    omega_slow = 0.0;
end

if ~Enable
    lambda_alpha1 = 0.0;
    lambda_beta1 = 0.0;
    lambda_alpha_hat = 0.0;
    lambda_beta_hat = 0.0;
    dhat_alpha = 0.0;
    dhat_beta = 0.0;
    theta_fast = 0.0;
    theta_slow = 0.0;
    omega_fast = 0.0;
    omega_slow = 0.0;
    pos_pu = single(0.0);
    speed_pu = single(0.0);
    lambda_alpha1_out = single(0.0);
    lambda_beta1_out = single(0.0);
    lambda_alpha2_out = single(0.0);
    lambda_beta2_out = single(0.0);
    dhat_alpha_out = single(0.0);
    dhat_beta_out = single(0.0);
    omega_fast_out = single(0.0);
    omega_slow_out = single(0.0);
    kdf_mode = false;
    kaf_mode = false;
    flux_limited = false;
    kdf_effective = single(0.0);
    test_bias_active = false;
    rotor_flux_mag = single(0.0);
    return;
end

v_alpha = double(VI_fb(1))*v_base;
v_beta = double(VI_fb(2))*v_base;
i_alpha = double(VI_fb(3))*i_base;
i_beta = double(VI_fb(4))*i_base;

if enable_voltage_preprocess
    v_alpha = v_alpha + v_alpha_preprocess;
    v_beta = v_beta + v_beta_preprocess;
end

% Inject only after the normal preprocessing hook and only in test mode.
test_bias_active = false;
if test_profile_enable && fado_test_vector(1) ~= 0
    v_alpha = v_alpha + double(fado_test_vector(2));
    v_beta = v_beta + double(fado_test_vector(3));
    test_bias_active = true;
end

rs_est = rs_nom*rs_scale;
lq_est = lq_nom*lq_scale;
omega_threshold = 2*pi*low_speed_hz;
kaf_mode = abs(omega_fast) <= omega_threshold;
kdf_mode = ~kaf_mode;
flux_limited = false;

kdf_command = kdf;
if test_profile_enable && fado_test_vector(4) ~= 0
    kdf_command = double(fado_test_vector(5));
end

rotor_flux_alpha = lambda_alpha1 - dhat_alpha - lq_est*i_alpha;
rotor_flux_beta = lambda_beta1 - dhat_beta - lq_est*i_beta;
rotor_flux_mag_si = hypot(rotor_flux_alpha, rotor_flux_beta);
if kaf_mode
    rotor_flux_alpha_limited = rotor_flux_alpha;
    rotor_flux_beta_limited = rotor_flux_beta;
    if rotor_flux_mag_si > flux_limit
        limiter_scale = flux_limit/rotor_flux_mag_si;
        rotor_flux_alpha_limited = rotor_flux_alpha*limiter_scale;
        rotor_flux_beta_limited = rotor_flux_beta*limiter_scale;
        flux_limited = true;
    end
    lambda_alpha_dot = v_alpha - rs_est*i_alpha - kaf*(rotor_flux_alpha - rotor_flux_alpha_limited);
    lambda_beta_dot = v_beta - rs_est*i_beta - kaf*(rotor_flux_beta - rotor_flux_beta_limited);
    kdf_effective = 0.0;
else
    kdf_effective = kdf_command;
    lambda_alpha_dot = v_alpha - rs_est*i_alpha - kdf_effective*dhat_alpha;
    lambda_beta_dot = v_beta - rs_est*i_beta - kdf_effective*dhat_beta;
end
lambda_alpha1 = lambda_alpha1 + Ts_fado*lambda_alpha_dot;
lambda_beta1 = lambda_beta1 + Ts_fado*lambda_beta_dot;

abs_omega = abs(omega_fast);
p1 = 2*abs_omega;
p2 = -omega_fast;
p3 = omega_fast;
p4 = 2*abs_omega;
q1 = 0.0;
q2 = -omega_fast;
q3 = omega_fast;
q4 = 0.0;
innovation_alpha = lambda_alpha1 - lambda_alpha_hat;
innovation_beta = lambda_beta1 - lambda_beta_hat;
lambda_alpha_hat_dot = -omega_fast*lambda_beta_hat + omega_fast*dhat_beta + p1*innovation_alpha + p2*innovation_beta;
lambda_beta_hat_dot = omega_fast*lambda_alpha_hat - omega_fast*dhat_alpha + p3*innovation_alpha + p4*innovation_beta;
dhat_alpha_dot = q1*innovation_alpha + q2*innovation_beta;
dhat_beta_dot = q3*innovation_alpha + q4*innovation_beta;
lambda_alpha_hat = lambda_alpha_hat + Ts_fado*lambda_alpha_hat_dot;
lambda_beta_hat = lambda_beta_hat + Ts_fado*lambda_beta_hat_dot;
dhat_alpha = dhat_alpha + Ts_fado*dhat_alpha_dot;
dhat_beta = dhat_beta + Ts_fado*dhat_beta_dot;

lambda_alpha2 = lambda_alpha1 - dhat_alpha;
lambda_beta2 = lambda_beta1 - dhat_beta;
theta_direct = atan2(lambda_beta2 - lq_est*i_beta, lambda_alpha2 - lq_est*i_alpha);

wn_fast = 2*pi*fast_bandwidth_hz;
phase_error_fast = fado_wrap_to_pi(theta_direct - theta_fast);
omega_fast = omega_fast + Ts_fado*wn_fast*wn_fast*phase_error_fast;
theta_fast = fado_wrap_to_pi(theta_fast + Ts_fado*(omega_fast + 2*zeta*wn_fast*phase_error_fast));

wn_slow = 2*pi*slow_bandwidth_hz;
phase_error_slow = fado_wrap_to_pi(theta_direct - theta_slow);
omega_slow = omega_slow + Ts_fado*wn_slow*wn_slow*phase_error_slow;
theta_slow = fado_wrap_to_pi(theta_slow + Ts_fado*(omega_slow + 2*zeta*wn_slow*phase_error_slow));

pos_pu = single(mod(theta_fast, 2*pi)/(2*pi));
speed_pu = single(omega_slow/(2*pi*pole_pairs)*(60/n_base));
lambda_alpha1_out = single(lambda_alpha1);
lambda_beta1_out = single(lambda_beta1);
lambda_alpha2_out = single(lambda_alpha2);
lambda_beta2_out = single(lambda_beta2);
dhat_alpha_out = single(dhat_alpha);
dhat_beta_out = single(dhat_beta);
omega_fast_out = single(omega_fast);
omega_slow_out = single(omega_slow);
kdf_effective = single(kdf_effective);
rotor_flux_mag = single(rotor_flux_mag_si);
end

function angle_out = fado_wrap_to_pi(angle_in)
angle_out = mod(angle_in + pi, 2*pi) - pi;
end

== matlab function mcb_pmsm_foc_sensorless_f28379d1/FADO_Id_Assist ==
  data: id_base_pu input single size=1; id_ref_pu output single size=1; iq_ref_pu input single size=1; estimator_selector input uint32 size=1; en_closed_loop input boolean size=1; low_speed_mode input boolean size=1; active output boolean size=1; enable_id_assist input single size=1; imin_pu input single size=1
function [id_ref_pu, active] = FADO_Id_Assist(id_base_pu, iq_ref_pu, estimator_selector, en_closed_loop, low_speed_mode, enable_id_assist, imin_pu)
id_ref_pu = id_base_pu;
active = false;
if estimator_selector == uint32(3) && en_closed_loop && low_speed_mode && enable_id_assist ~= 0
    id_ref_pu = single(sqrt(max(double(imin_pu)*double(imin_pu) - double(iq_ref_pu)*double(iq_ref_pu), 0)));
    active = true;
end
end
